simulink model "onlyDiscrete"  (R2021a)
settings: Solver=VariableStepAuto  StartTime=0.0  StopTime=10.0  RelTol=1e-3
undefined symbols (not defined in the file): cd_poly, denum_d, num_d, rd0, rd1, rd2, rd_poly, tc, Tq
settings Model: Creator=akangmufti  LastModifiedBy=akangmufti

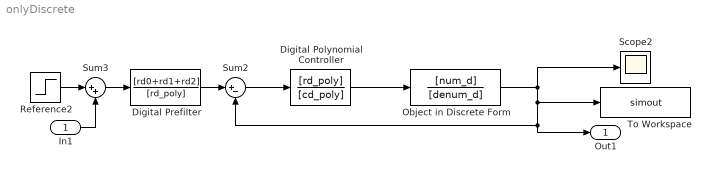
== system onlyDiscrete ==
  In1 : Inport
  Digital Polynomial Controller : DiscreteFilter  Numerator=[rd_poly]  Denominator=[cd_poly]  SampleTime=Tq
  Digital Prefilter : DiscreteFilter  Numerator=[rd0+rd1+rd2]  Denominator=[rd_poly]  SampleTime=Tq
  Object in Discrete Form : DiscreteTransferFcn  Numerator=[num_d]  Denominator=[denum_d]  SampleTime=Tq
  Reference2 : Step  Time=tc  SampleTime=0
  Scope2 : Scope
  Sum2 : Sum  Inputs=|+-
  Sum3 : Sum  Inputs=|++
  To Workspace : ToWorkspace  VariableName=simout  SampleTime=-1
  Out1 : Outport
  wires:
  Object in Discrete Form/1 -> To Workspace/1, Out1/1, Sum2/2, Scope2/1
  Sum3/1 -> Digital Prefilter/1
  Digital Prefilter/1 -> Sum2/1
  Sum2/1 -> Digital Polynomial Controller/1
  In1/1 -> Sum3/2
  Reference2/1 -> Sum3/1
  Digital Polynomial Controller/1 -> Object in Discrete Form/1
